simulink model "Traffic_Light_cs"  (R2019b)
settings: Solver=ode5  StartTime=0.0  StopTime=200  FixedStep=1/1000  RelTol=1e-3
PreLoadFcn:
  | mbxruntime.callbacks.PreLoadFcn(bdroot);
PostLoadFcn:
  | mbxruntime.callbacks.PostLoadFcn(bdroot);
InitFcn:
  | mbxruntime.callbacks.InitFcn(bdroot);
StartFcn:
  | mbxruntime.callbacks.StartFcn(bdroot);
StopFcn:
  | mbxruntime.callbacks.StopFcn(bdroot);
model workspace (MAT data in the model file):
  mbox_table : object (value not decoded)
  model_closed = 0
  sim_status = 0
values from neighbouring files (symbols this model uses):
  load_x1 = [-876.8956 -876.745665143 -876.595730285 -876.445795428 -876.29586057 -876.145925713 -875.995990855 -875.846055998 -875.69612114 -875.546186283 -875.396251425 -875.246316568 ... (5741 elements, 5741x1)]    [Data_ckx.mat]    (also in Load.mat)
  load_y1 = [537.3585 537.354079761 537.349659522 537.345239282 537.340819043 537.336398804 537.331978565 537.327558325 537.323138086 537.318717847 537.314297608 537.309877368 ... (5741 elements, 5741x1)]    [Data_ckx.mat]    (also in Load.mat)
  load_z1 = [0 0 0 0 0 0 0 0 0 0 0 0 ... (5741 elements, 5741x1)]    [Data_ckx.mat]    (also in Load.mat)
  q_pass = [0 0 0 37.0489514481 49.8894252687 51.0913174965 61.791576133 65.4762304223 75.669686677 80.4628164105 88.6197377629 94.2384891559 ... (437675 elements, 87535x5)]    [Data_ckx.mat]
  q_stop = [0 0 0 15.0544571491 15.7911831418 16.0935138936 18.6666396431 19.4721381181 21.7098800606 22.5642135149 25.0883481215 26.1253405703 ... (437675 elements, 87535x5)]    [Data_ckx.mat]
  s = roadinf.s    [Constraint_T_V.m]    (also in Light_Distinguish_old.m = 75:-0.7:75-84*0.7)
undefined symbols (not defined in the file or in its folder): InitImageOutputDir, mbxruntime, sigbuilder_block, tabledata
libraries: simulink x10, PreScanSimulinkLibrary x8, simulink_extras x4, autolibshared x1, fuzblock x1
(part 2 of 5)

== system Traffic_Light_cs/Synchronizer ==
  Bus Selector1 : BusSelector  OutputSignals=FederateStopped
  Stop Simulation : Stop
  sfun_Synchronizer : S-Function  FunctionName=sfun_Synchronizer  Parameters=SampleTime  SFunctionDeploymentMode=off  EnableBusSupport=off  mask(Legacy Function){SFunctionSpec=void prescan_synchronizer_outputFcn(void ** work1, PRESCAN_SYNCHRONIZEDATA y1[1]), SampleTime=TimeStep, ShowSpec=on}
      mask prompts: SampleTime "Sample time (-1 for inherited):"; ShowSpec "Display function specification"
      mask help:
      | This block allows you to call the legacy functions specified by the following Legacy Code Tool definition:
      | def.SFunctionName = 'sfun_Synchronizer';
      | def.OutputFcnSpec = 'void prescan_synchronizer_outputFcn(void ** work1, PRESCAN_SYNCHRONIZEDATA y1[1])';
      | def.StartFcnSpec = 'void prescan_synchronizer_startFcn(void ** work1)';
      | def.TerminateFcnSpec = 'void prescan_synchronizer_terminateFcn(void ** work1)';
      | def.HeaderFiles = {'prescan_synchronizer_data.h'};
      | def.HostLibFiles = {'sensorinterfaced.lib'};
      | def.IncPaths = {'src', 'C:\prescandev\vislibrary\vis\..\pimp\include\sensors\InterfaceRTW'};
      | def.SrcPaths = {'src'};
      | def.LibPaths = {'C:\\prescandev\\vislibrary_build\lib'};
      | def.SampleTime = 'parameterized';
      | def.Options.language = 'C';
      mask Help: <p>This block was generated automatically by the Legacy Code Tool. For detailed help on this tool, call<a href="matlab:legacy_code('help')"> legacy_code('help')</a>.</p>
      mask Callback ShowSpec:
      | if strcmp(get_param(gcbh, 'ShowSpec'), 'on')
      |   set_param(gcbh, 'MaskDisplay', sprintf('fprintf(''%s'');', get_param(gcbh, 'SFunctionSpec')));
      | else
      |   set_param(gcbh, 'MaskDisplay', sprintf('fprintf(''%s'');', get_param(gcbh, 'FunctionName')));
      | end
      mask Display: fprintf('void prescan_synchronizer_outputFcn(void ** work1, PRESCAN_SYNCHRONIZEDATA y1[1])');
  wires:
  Bus Selector1/1 -> Stop Simulation/1  "<FederateStopped>"
  sfun_Synchronizer/1 -> Bus Selector1/1

== system Traffic_Light_cs/VISUCasingLights_ID_1 ==
  VISUCasingLights_ID_1 : Inport  Tag=inport/VisuCasingLights  SampleTime=1/1000  BusOutputAsStruct=on
  Actuator : Subsystem  mask(PreScan Sink Block: VisuTrafficLight){UniqueID=35, ColorsObjectQuery=, Colors=[]}
      mask prompts: UniqueID "Parent Unique Identifier"; ColorsObjectQuery "Query for Color Object"; Colors "Matrix of colors"
      mask help:
      | The VisuTrafficLight block provides a way to animate traffic lights: switch on and off individual lights.
      |
      | For more information, please click Help.
      mask Help: eval('openHelp(731)')
      mask Display: image(imread('TrafficLightCasing.png'))
  wires:
  VISUCasingLights_ID_1/1 -> Actuator/1(VISUCasingLights_ID_1)

== system Traffic_Light_cs/VISUCasingLights_ID_2 ==
  VISUCasingLights_ID_2 : Inport  Tag=inport/VisuCasingLights  SampleTime=1/1000  BusOutputAsStruct=on
  Actuator : Subsystem  mask(PreScan Sink Block: VisuTrafficLight){UniqueID=525, ColorsObjectQuery=, Colors=[]}
      mask prompts: UniqueID "Parent Unique Identifier"; ColorsObjectQuery "Query for Color Object"; Colors "Matrix of colors"
      mask help:
      | The VisuTrafficLight block provides a way to animate traffic lights: switch on and off individual lights.
      |
      | For more information, please click Help.
      mask Help: eval('openHelp(731)')
      mask Display: image(imread('TrafficLightCasing.png'))
  wires:
  VISUCasingLights_ID_2/1 -> Actuator/1(VISUCasingLights_ID_2)

== system Traffic_Light_cs/VISUCasingLights_ID_3 ==
  VISUCasingLights_ID_3 : Inport  Tag=inport/VisuCasingLights  SampleTime=1/1000  BusOutputAsStruct=on
  Actuator : Subsystem  mask(PreScan Sink Block: VisuTrafficLight){UniqueID=526, ColorsObjectQuery=, Colors=[]}
      mask prompts: UniqueID "Parent Unique Identifier"; ColorsObjectQuery "Query for Color Object"; Colors "Matrix of colors"
      mask help:
      | The VisuTrafficLight block provides a way to animate traffic lights: switch on and off individual lights.
      |
      | For more information, please click Help.
      mask Help: eval('openHelp(731)')
      mask Display: image(imread('TrafficLightCasing.png'))
  wires:
  VISUCasingLights_ID_3/1 -> Actuator/1(VISUCasingLights_ID_3)

== system Traffic_Light_cs/CAR_Ahead/CameraSensor_2_CM_Demux ==
  In1 : Inport
  Selector : Selector  NumberOfDimensions=2  InputPortWidth=3  IndexOptions=Index vector (dialog),Index vector (dialog)  Indices=-1,1:hres  OutputSizes=1,1
  Selector1 : Selector  NumberOfDimensions=2  InputPortWidth=3  IndexOptions=Index vector (dialog),Index vector (dialog)  Indices=-1,hres+1:hres*2  OutputSizes=1,1
  Selector2 : Selector  NumberOfDimensions=2  InputPortWidth=3  IndexOptions=Index vector (dialog),Index vector (dialog)  Indices=-1,hres*2+1:hres*3  OutputSizes=1,1
  R : Outport
  G : Outport  Port=2
  B : Outport  Port=3
  wires:
  In1/1 -> Selector1/1, Selector/1, Selector2/1
  Selector/1 -> R/1
  Selector1/1 -> G/1
  Selector2/1 -> B/1

== system Traffic_Light_cs/CAR_Ahead/Decision ==
  Dis_Car2Light_Ahead : Inport
  CameraSensor_Ahead : Inport  Port=2
  Traffic_State : Inport  Port=3
  Traffic_Time : Inport  Port=4
  TrafficLight_ID_Ahead : Inport  Port=5
  PhaseTime : Inport  Tag=inport/SelfPort  Port=6  SampleTime=1/20  BusOutputAsStruct=on
  V_now : Inport  Port=7
  traffic_state : Inport  Port=8
  Bus Selector : BusSelector  OutputSignals=ID1,ID2,ID3
  Chart : Stateflow chart  TreatAsAtomicUnit=on
  Function-Call Subsystem : Subsystem  TreatAsAtomicUnit=on
  Multiport Switch : MultiPortSwitch  DiagnosticForDefault=None
  Light_State_Ahead : Outport  VectorParamsAs1DForOutWhenUnconnected=off
  TrafficLight_PhaseTime : Outport  Port=2  VectorParamsAs1DForOutWhenUnconnected=off
  wires:
  V_now/1 -> Function-Call Subsystem/5(V_now)
  Traffic_Time/1 -> Function-Call Subsystem/4(Traffic_Time)
  TrafficLight_ID_Ahead/1 -> Function-Call Subsystem/7(TrafficLight_ID_Ahead), Multiport Switch/1
  Chart/1(Decision_Call()) -> Function-Call Subsystem/Trigger
  Bus Selector/1 -> Multiport Switch/2  "<ID1>"
  Traffic_State/1 -> Function-Call Subsystem/3(Traffic_State)
  Bus Selector/2 -> Multiport Switch/3  "<ID2>"
  Function-Call Subsystem/1(Light_State_Ahead) -> Light_State_Ahead/1
  Bus Selector/3 -> Multiport Switch/4  "<ID3>"
  CameraSensor_Ahead/1 -> Function-Call Subsystem/2("CameraSensor ")
  Dis_Car2Light_Ahead/1 -> Chart/1(Dis_Car2Light_0919_100), Function-Call Subsystem/1(Dis)
  Multiport Switch/1 -> TrafficLight_PhaseTime/1
  PhaseTime/1 -> Bus Selector/1
  traffic_state/1 -> Function-Call Subsystem/6(traffic_state)

== system Traffic_Light_cs/CAR_Ahead/SELF_Demux ==
  SELF : Inport  OutDataTypeStr=Bus: PRESCAN_SELFSENSORDATA
  Bus Selector : BusSelector  OutputSignals=PositionX,PositionY,PositionZ,OrientationRoll,OrientationPitch,OrientationYaw,Velocity,Yaw_rate,Lat,Long,Alt
  Demux2 : Demux  Outputs=3
  Gain : Gain  Gain=180/pi
  Gain1 : Gain  Gain=180/pi
  Vector Concatenate1 : Concatenate  NumInputs=3
  compas converter : Subsystem
  x [m] : Outport
  y [m] : Outport  Port=2
  z [m] : Outport  Port=3
  rotx [deg] : Outport  Port=4
  roty [deg] : Outport  Port=5
  rotz [deg] : Outport  Port=6
  GPS lat [deg] : Outport  Port=7
  GPS long [deg] : Outport  Port=8
  GPS alt [m] : Outport  Port=9
  velocity [m/s] : Outport  Port=10
  heading [deg] : Outport  Port=11
  yaw rate [deg/s] : Outport  Port=12
  wires:
  Bus Selector/11 -> GPS alt [m]/1  "<Alt>"
  Bus Selector/10 -> GPS long [deg]/1  "<Long>"
  Bus Selector/9 -> GPS lat [deg]/1  "<Lat>"
  Bus Selector/8 -> Gain1/1  "<Yaw_rate>"
  Bus Selector/7 -> velocity [m/s]/1  "<Velocity>"
  Bus Selector/6 -> compas converter/1(rotz [rad]), Vector Concatenate1/3  "<OrientationYaw>"
  Bus Selector/5 -> Vector Concatenate1/2  "<OrientationPitch>"
  Bus Selector/4 -> Vector Concatenate1/1  "<OrientationRoll>"
  Vector Concatenate1/1 -> Gain/1
  Bus Selector/3 -> z [m]/1  "<PositionZ>"
  Bus Selector/2 -> y [m]/1  "<PositionY>"
  Bus Selector/1 -> x [m]/1  "<PositionX>"
  SELF/1 -> Bus Selector/1
  Gain/1 -> Demux2/1
  Demux2/1 -> rotx [deg]/1
  Demux2/2 -> roty [deg]/1
  Demux2/3 -> rotz [deg]/1
  compas converter/1(heading [deg]) -> heading [deg]/1
  Gain1/1 -> yaw rate [deg/s]/1

== system Traffic_Light_cs/CAR_Ahead/STATE_CAR_Ahead ==
  State : Inport  SampleTime=TimeStep
  Bus Creator : BusCreator  Inputs=15  OutDataTypeStr=Bus: PRESCAN_STATEACTUATORDATA  NonVirtualBus=on
  Demux : Demux  Outputs=15
  iniBODYAngles wrtVEH [rad] : Constant  Value=[Roll0 Pitch0 0]  SampleTime=TimeStep
  iniVEHAngles wrtGLOB [rad] : Constant  Value=[0 0 Yaw0]  SampleTime=TimeStep
  iniVEHposition wrtGLOB [m] : Constant  Value=[x0 y0 z0]  SampleTime=TimeStep
  state2FullState : PreScanSimulinkLibrary/state2FullState  SystemSampleTime=-1  Latency=0  AutoFrameSizeCalculation=off
  StateBus : Outport  OutDataTypeStr=Bus: PRESCAN_STATEACTUATORDATA
  wires:
  Bus Creator/1 -> StateBus/1
  State/1 -> state2FullState/1
  state2FullState/1 -> Demux/1
  iniVEHposition wrtGLOB [m]/1 -> state2FullState/2
  iniBODYAngles wrtVEH [rad]/1 -> state2FullState/3
  iniVEHAngles wrtGLOB [rad]/1 -> state2FullState/4
  Demux/1 -> Bus Creator/1  "PositionX"
  Demux/2 -> Bus Creator/2  "PositionY"
  Demux/3 -> Bus Creator/3  "PositionZ"
  Demux/4 -> Bus Creator/4  "VelocityX"
  Demux/5 -> Bus Creator/5  "VelocityY"
  Demux/6 -> Bus Creator/6  "VelocityZ"
  Demux/7 -> Bus Creator/7  "AccelerationX"
  Demux/8 -> Bus Creator/8  "AccelerationY"
  Demux/9 -> Bus Creator/9  "AccelerationZ"
  Demux/10 -> Bus Creator/10  "OrientationRoll"
  Demux/11 -> Bus Creator/11  "OrientationPitch"
  Demux/12 -> Bus Creator/12  "OrientationYaw"
  Demux/13 -> Bus Creator/13  "AngularVelocityRoll"
  Demux/14 -> Bus Creator/14  "AngularVelocityPitch"
  Demux/15 -> Bus Creator/15  "AngularVelocityYaw"

== system Traffic_Light_cs/CAR_Ahead/Subsystem ==
  x [m] : Inport
  y [m] : Inport  Port=2
  Bus Creator : BusCreator  Inputs=6
  Bus Creator1 : BusCreator  Inputs=4
  Delay : Delay
  Delay1 : Delay
  MATLAB Function : MATLAB Function  TreatAsAtomicUnit=on
  Signal Builder : Subsystem  Tag=STV Subsys  LoadFcn=sigbuilder_block('load');  StartFcn=sigbuilder_block('start');  StopFcn=sigbuilder_block('stop');  ClipboardFcn=sigbuilder_block('clipboard');  mask(Sigbuilder block){tuvar=[0:10]}
      mask help: Simulink:masks:SigbuilderBlock_MD
      mask init:
      | if ~strcmp(get_param(bdroot(gcbh),'SimulationStatus'),'stopped') tuvar = sigbuilder_block('maskInit'); end
      settings: CopyFcn=sigbuilder_block('copy');  DeleteFcn=sigbuilder_block('delete');  ModelCloseFcn=sigbuilder_block('modelClose');  PreSaveFcn=sigbuilder_block('preSave');  PauseFcn=sigbuilder_block('pause');  ContinueFcn=sigbuilder_block('continue');  NameChangeFcn=sigbuilder_block('namechange');  OpenFcn=sigbuilder_block('open',[6 6 1188 604.5 ]);  CloseFcn=sigbuilder_block('close');
      mask Display: plot(0, 0, 100, 100,[2, 2, 32, 32, 2], [68, 8, 8, 68, 68],[32, 2], [38, 38], [32, 19, 2],[53, 60, 44], [32, 17, 17, 2],[16, 16, 31, 31]);txt = getActiveGroup(gcbh);text(2, 100, txt,'verticalAlignment', 'top');
  Distance2Light : Outport  VectorParamsAs1DForOutWhenUnconnected=off
  TrafficLight_ID : Outport  Port=2  VectorParamsAs1DForOutWhenUnconnected=off
  wires:
  MATLAB Function/2(Dis_Car2Light) -> Distance2Light/1  "Dis_Car2Light"
  Bus Creator1/1 -> MATLAB Function/1(Car_GPS)
  Delay/1 -> Bus Creator1/3
  Delay1/1 -> Bus Creator1/1
  MATLAB Function/1(TrafficLight_ID) -> TrafficLight_ID/1  "TrafficLight_ID"
  Bus Creator/1 -> MATLAB Function/2(TrafficLight_GPS)
  Signal Builder/6(ID==3,Y) -> Bus Creator/6
  Signal Builder/5(ID==3,X) -> Bus Creator/5
  Signal Builder/4(ID==2,Y) -> Bus Creator/4
  Signal Builder/3(ID==2,X) -> Bus Creator/3
  Signal Builder/2(ID==1,Y) -> Bus Creator/2
  Signal Builder/1(ID==1,X) -> Bus Creator/1
  y [m]/1 -> Bus Creator1/4, Delay/1
  x [m]/1 -> Bus Creator1/2, Delay1/1

== system Traffic_Light_cs/CAR_Ahead/Trajectories ==
  Traj2State1 : Subsystem  Tag=Traj2State  mask(PreScan Demux Block:){}
      settings: DeleteFcn=PreScanBlockDeleteFcn;
  TrajCoGOffset : Subsystem  Tag=TrajCoGOffset  mask(Trajectory CoG Offset block){CoGOffsetZ=0.55, InitRoll=0, InitPitch=0}
      mask prompts: CoGOffsetZ "Z-component of CoG Offset [m]:"; InitRoll "Initial Roll angle [deg]:"; InitPitch "Initial Pitch angle [deg]:"
      mask help: A trajectory follows the surface of the road. However the position of a actor is based on the actor's Center of Gravity, which is typically above the road. This block converts from the trajectory along the road surface to the trajectory of the actor's CoG by realigning the z-component of the CoG offset to be normal to the road.
      settings: DeleteFcn=PreScanBlockDeleteFcn;
  Trajectory_1 : Subsystem  Tag=Trajectory  mask(PreScan Source Block: Trajectory){FileName='Trajectory_1.mat', TimeStep=1/1000}
      mask prompts: TimeStep "Time Step [s]"
      mask help:
      | The Trajectory block contains the trajectories defined in the PreScan Experiment Editor. The output of the trajectory block is the (vehicle) State.
      |
      | For more information, please click Help.
      mask init:
      | EXPROOT=pwd;  % TODO better construction for locating base experiment
      | 
      | trajfilename = fullfile(EXPROOT,'Trajectories',FileName);
      | load(trajfilename);
      | trajectory=trajectory';
      | 
      | traj.time=trajectory(:,1);%[];
      | traj.signals.values=trajectory(:,2:19);
      | traj.dimensions=18;
      | traj.label='';
      | 
      | SampleTime=traj.time(2)-traj.time(1);
      settings: DeleteFcn=PreScanBlockDeleteFcn;
      mask Help: eval('openHelp(312)')
      mask Display: fprintf(FileName)
  Trajectory_1_Offset : Constant  Tag=TrajectoryOffset  Value="[0  0  0  0  0  0]"
  State : Outport  Tag=TrajOutport
  wires:
  Trajectory_1/1(trajectory) -> Traj2State1/1(Traj Org)
  Trajectory_1_Offset/1 -> Traj2State1/2(Offset)
  TrajCoGOffset/1(State Out) -> State/1
  Traj2State1/1(state) -> TrajCoGOffset/1(State In)

== system Traffic_Light_cs/CAR_Ahead/V2V_Output ==
  Traffic_State : Inport
  Dis_Car2Light_Ahead : Inport  Port=2
  Light_State_Ahead : Inport  Port=3
  TrafficLight_ID_Ahead : Inport  Port=4
  Traffic_Time : Inport  Port=5
  TrafficLight_PhaseTime : Inport  Port=6
  Bus Creator : BusCreator  Inputs=3
  Switch : Switch  Criteria=u2 > Threshold
  Switch1 : Switch  Criteria=u2 > Threshold  Threshold=500
  Traffic_Information : Outport  VectorParamsAs1DForOutWhenUnconnected=off
  "Traffic_Time " : Outport  Port=2  VectorParamsAs1DForOutWhenUnconnected=off
  wires:
  Light_State_Ahead/1 -> Switch1/3
  Bus Creator/1 -> Traffic_Information/1
  Traffic_State/1 -> Switch1/1
  TrafficLight_PhaseTime/1 -> Switch/3
  Switch1/1 -> Bus Creator/1  "LightState_Ahead"
  TrafficLight_ID_Ahead/1 -> Bus Creator/2  "ID_Ahead"
  Traffic_Time/1 -> Switch/1, Switch/2
  Dis_Car2Light_Ahead/1 -> Switch1/2
  Switch/1 -> Bus Creator/3, "Traffic_Time "/1  "TrafficTime_Ahead"

== system Traffic_Light_cs/CAR_Main/CameraSensor_1_CM_Demux ==
  In1 : Inport
  Selector : Selector  NumberOfDimensions=2  InputPortWidth=3  IndexOptions=Index vector (dialog),Index vector (dialog)  Indices=-1,1:hres  OutputSizes=1,1
  Selector1 : Selector  NumberOfDimensions=2  InputPortWidth=3  IndexOptions=Index vector (dialog),Index vector (dialog)  Indices=-1,hres+1:hres*2  OutputSizes=1,1
  Selector2 : Selector  NumberOfDimensions=2  InputPortWidth=3  IndexOptions=Index vector (dialog),Index vector (dialog)  Indices=-1,hres*2+1:hres*3  OutputSizes=1,1
  R : Outport
  G : Outport  Port=2
  B : Outport  Port=3
  wires:
  In1/1 -> Selector1/1, Selector/1, Selector2/1
  Selector/1 -> R/1
  Selector1/1 -> G/1
  Selector2/1 -> B/1

== system Traffic_Light_cs/CAR_Main/Decision ==
  Dis_Car2Light_Main : Inport
  CameraSensor_Main : Inport  Port=2
  Traffic_State : Inport  Port=3
  Traffic_Time : Inport  Port=4
  TrafficLight_ID_Main : Inport  Port=5
  PhaseTime : Inport  Tag=inport/SelfPort  Port=6  SampleTime=1/20  BusOutputAsStruct=on
  V_now : Inport  Port=7
  traffic_state : Inport  Port=8
  Bus Selector : BusSelector  OutputSignals=ID1,ID2,ID3
  Chart : Stateflow chart  TreatAsAtomicUnit=on
  Function-Call Subsystem : Subsystem  TreatAsAtomicUnit=on
  Multiport Switch : MultiPortSwitch  DiagnosticForDefault=None
  Switch : Switch  Criteria=u2 > Threshold  Threshold=-1
  Transfer Fcn : TransferFcn  Denominator=[4 1]
  Light_State_Main : Outport  VectorParamsAs1DForOutWhenUnconnected=off
  TrafficLight_PhaseTime : Outport  Port=2  VectorParamsAs1DForOutWhenUnconnected=off
  V_Target : Outport  Port=3  VectorParamsAs1DForOutWhenUnconnected=off
  wires:
  Transfer Fcn/1 -> Switch/3
  Function-Call Subsystem/2(V_Target) -> Switch/1, Transfer Fcn/1
  Switch/1 -> V_Target/1
  Function-Call Subsystem/3("Suggest ") -> Switch/2
  V_now/1 -> Function-Call Subsystem/5(V_now)
  Traffic_Time/1 -> Function-Call Subsystem/4(Traffic_Time)
  TrafficLight_ID_Main/1 -> Function-Call Subsystem/7(TrafficLight_ID_Main), Multiport Switch/1
  Chart/1(Decision_Call()) -> Function-Call Subsystem/Trigger
  Bus Selector/3 -> Multiport Switch/4  "<ID3>"
  Bus Selector/1 -> Multiport Switch/2  "<ID1>"
  Traffic_State/1 -> Function-Call Subsystem/3(Traffic_State)
  Bus Selector/2 -> Multiport Switch/3  "<ID2>"
  Function-Call Subsystem/1(Light_State_Main) -> Light_State_Main/1
  CameraSensor_Main/1 -> Function-Call Subsystem/2("CameraSensor ")
  Dis_Car2Light_Main/1 -> Chart/1(Dis_Car2Light_0919_100), Function-Call Subsystem/1(Dis)
  Multiport Switch/1 -> TrafficLight_PhaseTime/1
  PhaseTime/1 -> Bus Selector/1
  traffic_state/1 -> Function-Call Subsystem/6(traffic_state)

== system Traffic_Light_cs/CAR_Main/Driver Model ==
  VehSpdTarKph : Inport
  VehSpdActKph : Inport  Port=2
  Grade[deg] : Inport  Port=3
  Abs : Abs
  Compare To Constant : simulink/Logic and Bit Operations/Compare To Constant  relop=<=  const=2/3.6  OutDataTypeStr=boolean
  Compare To Zero : simulink/Logic and Bit Operations/Compare To Zero  relop===  OutDataTypeStr=boolean
  Compare To Zero2 : simulink/Logic and Bit Operations/Compare To Zero  relop=>=  OutDataTypeStr=boolean
  Constant : Constant  Value=20
  D : Constant  Value=3
  Gain3 : Gain  Gain=100
  Gain4 : Gain  Gain=100
  Logical Operator : Logic  AllPortsSameDT=off  OutDataTypeStr=boolean
  Longitudinal Driver : autolibshared/Longitudinal Driver  cntrlType=PI  shftType=None  velUnits=m/s  gearOut=off  Kp=5  Ki=3  Kff=.01  Kg=.01  VehVelVec=[0 100]  KffVec=[.1 .1]  KpVec=[10 10]  KiVec=[5 5]  KgVec=[0 0]  m=1500  Kpt=3000  tau=.1  L=2  aR=200  bR=2.5  cR=.5  g=9.81  vnom=60  Kaw=.1  tauerr=.03  tauPt=2  GearInit=0  tShift=.1  pdlVec=[0.1 0.4 0.5 0.9]  upShftTbl=[-1 12.9375 26.4375 39.9375 51.18749999999999 62.4375 72.84375 83.25;-1 16.3125 29.8125 43.3125 54.5624 65.8125 76.78125 87.75;-1 19.6875 33.1875 46.68749999999999 57.9375 69.1875 80.71875 92.25;-1 33 52.5 77.25 100.5 138.75 161.875 185]  dwnShftTbl=[1 9.5625 23.0625 36.5625 47.8125 59.0625 68.90625 78.75;1 12.9375 26.4375 39.9375 51.18749999999999 62.4375 72.84375 83.25;1 16.3125 29.8125 43.3125 54.562499 65.8125 76.78125 87.75;1 19.6875 33.1875 46.68749999999999 57.9375 69.1875 80.71875 92.25]  tClutch=.5  tRev=.5  tPark=120  aMode=1  UpGearVec="[0  1  2  3  4  5  6  7]"  DownGearVec="[1  2  3  4  5  6  7  8]"
      settings: SourceProductBaseCode=PW
  N : Constant  Value=2
  R : Constant
  Relational Operator : RelationalOperator  Operator=~=  OutDataTypeStr=boolean  RndMeth=Simplest
  Subtract : Sum  Inputs=+-
  Switch1 : Switch  Criteria=u2 > Threshold
  Switch2 : Switch  Criteria=u2 > Threshold
  Switch3 : Switch  Criteria=u2 ~= 0
  Terminator : Terminator
  AccPedlRat% : Outport  VectorParamsAs1DForOutWhenUnconnected=off
  BrkPedlRat% : Outport  Port=2  VectorParamsAs1DForOutWhenUnconnected=off
  ShiftLvr : Outport  Port=3  VectorParamsAs1DForOutWhenUnconnected=off
  wires:
  Longitudinal Driver/1 -> Terminator/1
  Abs/1 -> Compare To Constant/1
  Subtract/1 -> Abs/1
  Constant/1 -> Switch3/3
  Gain4/1 -> Switch3/1  "BrkPedl"
  Relational Operator/1 -> Switch3/2
  R/1 -> Switch2/3
  Compare To Zero2/1 -> Switch2/2
  D/1 -> Switch2/1
  Compare To Constant/1 -> Logical Operator/2
  Compare To Zero/1 -> Logical Operator/1
  Logical Operator/1 -> Switch1/2
  Switch3/1 -> BrkPedlRat%/1  "BrkPedl"
  Longitudinal Driver/2 -> Gain3/1
  Longitudinal Driver/3 -> Gain4/1
  VehSpdTarKph/1 -> Compare To Zero/1, Compare To Zero2/1, Subtract/1, Longitudinal Driver/1
  Grade[deg]/1 -> Longitudinal Driver/3
  VehSpdActKph/1 -> Subtract/2, Longitudinal Driver/2
  Switch2/1 -> Switch1/3
  Switch1/1 -> ShiftLvr/1, Relational Operator/2
  N/1 -> Relational Operator/1, Switch1/1
  Gain3/1 -> AccPedlRat%/1  "AccPedl"

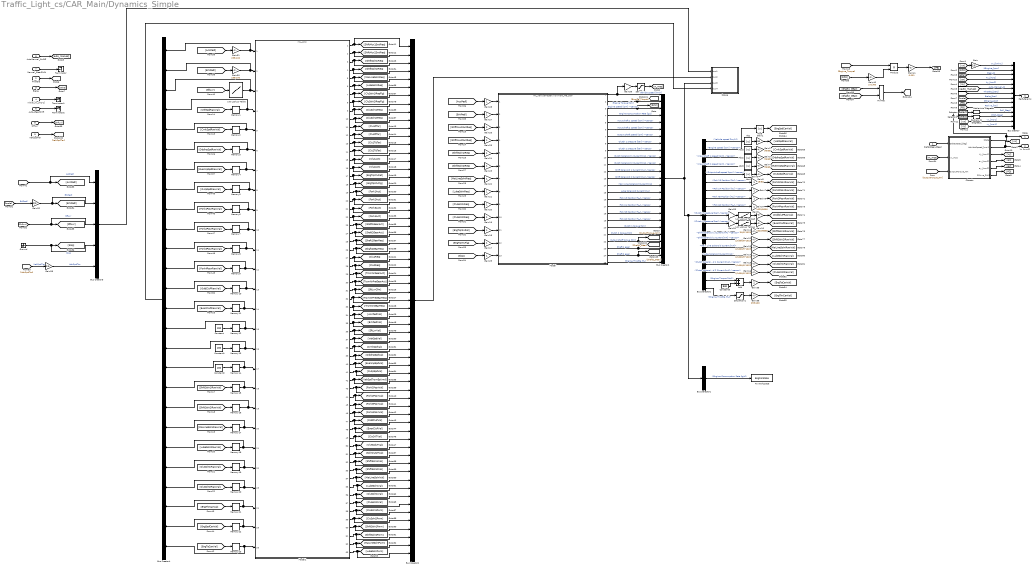
== system Traffic_Light_cs/CAR_Main/Dynamics_Simple ==
  DeltaSteer_[deg] : Inport
  Throttle : Inport  Port=2
  Brake : Inport  Port=3
  Initial_Vx_[ms-1] : Inport  Port=4
  AutoManual_OnOff : Inport  Port=5
  Auto_GearShift : Inport  Port=6
  Manual_GearShift : Inport  Port=7
  "ShfLvr " : Inport  Port=8
  "VehSpdTar " : Inport  Port=9
  1-D Lookup Table : Lookup_n-D  NumberOfTableDimensions=1  BreakpointsForDimension1=[0 1 2 3]  Table=[8 7 6 5]  TableDataTypeStr=uint8  InterpMethod=Flat  ExtrapMethod=Clip  DiagnosticForOutOfRangeInput=Warning  InternalRulePriority=Speed  OutDataTypeStr=uint8  RndMeth=Simplest  InputSameDT=on
  1-D Lookup Table1 : Lookup_n-D  NumberOfTableDimensions=1  BreakpointsForDimension1=[310,2500,20000]  Table=[0,500,4500]  TableDataTypeStr=Inherit: Inherit from 'Table data'  ExtrapMethod=Clip  UseLastTableValue=on  InternalRulePriority=Speed  OutDataTypeStr=Inherit: Inherit from 'Table data'  RndMeth=Simplest  InputSameDT=on
  1-D Lookup Table3 : Lookup_n-D  NumberOfTableDimensions=1  BreakpointsForDimension1=[310,2500,20000]  Table=[0,500,4500]  TableDataTypeStr=Inherit: Inherit from 'Table data'  ExtrapMethod=Clip  UseLastTableValue=on  InternalRulePriority=Speed  OutDataTypeStr=Inherit: Inherit from 'Table data'  RndMeth=Simplest  InputSameDT=on
  Abs{,1..4} (5 alike) : Abs
  Abs5 : Abs  OutDataTypeStr=uint16
  Add : Sum
  Bus Creator : BusCreator  Inputs=14
  Bus Creator1 : BusCreator  Inputs=25
  Bus Creator2 : BusCreator  Inputs=63
  Bus Creator3 : BusCreator  Inputs=5
  Bus Creator4 : BusCreator  Inputs=26
  Bus Selector1 : BusSelector  OutputSignals=Engine Consumption Rate [g/s]
  Bus Selector2 : BusSelector  OutputSignals=Vehicle speed [km/h],Engine speed [rpm] ->sensor,Input shaft 1 speed [rpm] ->sensor,Input shaft 2 speed [rpm] ->sensor,Output shaft speed [rpm] ->sensor,Fork 13 Position [‰] ->sensor,Fork 24 Position [‰] ->sensor,Fork N5 Position [‰] ->sensor,Fork 6R Position [‰] ->sensor,Clutch 1 pressure [bar] ->sensor,Clutch 2 pressure [bar] ->sensor,Shift Solenoid 1 Current [mA] ->sensor,Shift Solenoid 2 Current [mA] ->sensor,Main Line Solenoid Current [mA],Lube Solenoid Current [mA],Clutch Solenoid 1 Current [mA] ->sensor,Clutch Solenoid 2 Current [mA] ->sensor,Engine Torque [Nm],Engine Throttle [%]
  Chassis : Subsystem
      mask Display: image(imread('Chassis.png'));
  Constant : Constant  Value=200  OutDataTypeStr=uint16
  Constant1 : Constant  Value=200  OutDataTypeStr=uint16
  Constant2 : Constant  Value=200  OutDataTypeStr=uint16
  Constant3 : Constant  Value=848
  Gain : Gain  Gain=3.6
  Gain1 : Gain  Gain=64  OutDataTypeStr=uint16
  Gain10 : Gain  Gain=1023/5000  OutDataTypeStr=uint16
  Gain{11..16} (6 alike) : Gain  Gain=2/1000/5*1023  OutDataTypeStr=uint16
  Gain{17..29} (13 alike) : Gain  OutDataTypeStr=double
  Gain2 : Gain  Gain=36/60  OutDataTypeStr=uint16
  Gain3 : Gain  Gain=36/60  OutDataTypeStr=uint16
  Gain30 : Gain  Gain=255/100  OutDataTypeStr=uint8
  Gain31 : Gain  Gain=255/100  OutDataTypeStr=uint8
  Gain32 : Gain  Gain=2/3
  Gain33 : Gain  Gain=1000  OutDataTypeStr=uint16
  Gain34 : Gain  Gain=1000  OutDataTypeStr=uint16
  Gain35 : Gain  Gain=2  OutDataTypeStr=uint16
  Gain36 : Gain  Gain=255/100  OutDataTypeStr=uint8
  Gain37 : Gain  Gain=1023/5000  OutDataTypeStr=uint16
  Gain38 : Gain  Gain=3.6
  Gain39 : Gain  Gain=1/3.6
  Gain4 : Gain  Gain=36/60  OutDataTypeStr=uint16
  Gain40 : Gain  Gain=2*pi/60
  Gain41 : Gain  Gain=0.001
  Gain5 : Gain  Gain=18/60  OutDataTypeStr=uint16
  Gain{6..9} (4 alike) : Gain  OutDataTypeStr=uint16
  Ground : Ground
  Memory{1..23} (23 alike) : Memory  InheritSampleTime=on
  MinMax : MinMax  Function=max  Inputs=2
  Model : ModelReference  ModelNameDialog=MIL_VehicleTestEnvironment_MG_DCT.mdl  SimulationMode=Normal  ModelReferenceVersion=1.244
  Model1 : ModelReference  ModelNameDialog=MIL_ASW.slx  SimulationMode=Normal  ModelReferenceVersion=1.234
  Product : Product
  Radians to Degrees : simulink_extras/Transformations/Radians to Degrees
  Radians to Degrees1 : simulink_extras/Transformations/Radians to Degrees
  Saturation : Saturate  UpperLimit=20  LowerLimit=0
  Saturation1 : Saturate  UpperLimit=100  LowerLimit=0  OutDataTypeStr=double
  Scope : Subsystem
  Selector : Selector  InputPortWidth=9  IndexOptions=Index vector (dialog)  Indices=7  OutputSizes=1
  Selector1 : Selector  InputPortWidth=9  IndexOptions=Index vector (dialog)  Indices=8  OutputSizes=1
  Terminator : Terminator
  Terminator1 : Terminator
  Terminator2 : Terminator
  To Workspace : ToWorkspace  VariableName=EngConRate  SaveFormat=Timeseries  SampleTime=-1
  State : Outport  VectorParamsAs1DForOutWhenUnconnected=off
  Vx [m s-1] : Outport  Port=2  VectorParamsAs1DForOutWhenUnconnected=off
  Perf_Params : Outport  Port=3  VectorParamsAs1DForOutWhenUnconnected=off
  wires:
  Saturation/1 -> [vx_mps]
  Auto_GearShift/1 -> Terminator2/1
  Initial_Vx_[ms-1]/1 -> Terminator1/1
  Manual_GearShift/1 -> Terminator/1
  MinMax/1 -> [gear]
  [Shaft2_Gear] -> MinMax/2
  [Shaft1_Gear] -> MinMax/1
  Gain40/1 -> Product/2
  Gain41/1 -> [PE]
  [Engine_Torque] -> Product/1
  Product/1 -> Gain41/1
  [RPM] -> Gain40/1
  [OutputTorque_Nm] -> Chassis/3(OutputTorque_Nm)
  [vx_mps] -> Chassis/2(vx_mps)
  DeltaSteer_[deg]/1 -> Chassis/1(DeltaSteer_[deg])
  Brake/1 -> [brake]
  Throttle/1 -> [throttle]
  AutoManual_OnOff/1 -> [auto_manual]
  "ShfLvr "/1 -> [ShfLvr]
  "VehSpdTar "/1 -> [VehSpdTar]
  Gain39/1 -> Saturation/1
  Gain38/1 -> Bus Creator3/5  "VehSpdTar"
  Gain32/1 -> Bus Creator3/2, [BrkPedl]  "BrkPedl"
  Model/24 -> Bus Creator1/24, [Shaft2_Gear]  "Shaft 2 gear"
  Model/1 -> Gain39/1, Bus Creator1/1  "Vehicle speed [km/h]"
  Model/2 -> Bus Creator1/2, [Engine_Torque]  "Engine Torque [Nm]"
  Model/15 -> Bus Creator1/15  "Lube Solenoid Current [mA]"
  Model/23 -> Bus Creator1/23, [Shaft1_Gear]  "Shaft 1 gear"
  Model/19 -> Bus Creator1/19  "Fork 6R Position [‰] ->sensor"
  Model/5 -> Bus Creator1/5  "Input shaft 1 speed [rpm] ->sensor"
  Model/10 -> Bus Creator1/10  "Clutch Solenoid 1 Current [mA] ->sensor"
  Model/20 -> Bus Creator1/20  "Clutch 1 torque [Nm]"
  Model/9 -> Bus Creator1/9  "Clutch 2 pressure [bar] ->sensor"
  Model/3 -> Bus Creator1/3, [RPM]  "Engine speed [rpm] ->sensor"
  Model/14 -> Bus Creator1/14  "Main Line Solenoid Current [mA]"
  Model/12 -> Bus Creator1/12  "Shift Solenoid 1 Current [mA] ->sensor"
  Model/22 -> Bus Creator1/22, [OutputTorque_Nm]  "Output shaft torque [Nm]"
  Model/16 -> Bus Creator1/16  "Fork 13 Position [‰] ->sensor"
  Model/8 -> Bus Creator1/8  "Clutch 1 pressure [bar] ->sensor"
  Model/17 -> Bus Creator1/17  "Fork 24 Position [‰] ->sensor"
  Model/6 -> Bus Creator1/6  "Input shaft 2 speed [rpm] ->sensor"
  Model/11 -> Bus Creator1/11  "Clutch Solenoid 2 Current [mA] ->sensor"
  Model/13 -> Bus Creator1/13  "Shift Solenoid 2 Current [mA] ->sensor"
  Model/18 -> Bus Creator1/18  "Fork N5 Position [‰] ->sensor"
  Model/21 -> Bus Creator1/21  "Clutch 2 torque [Nm]"
  Model/7 -> Bus Creator1/7  "Output shaft speed [rpm] ->sensor"
  Model1/1 -> Bus Creator2/1, [ShiftMux1SwtReq]
  Model1/2 -> Bus Creator2/2, [ShiftMux2SwtReq]
  Model1/20 -> Bus Creator2/20, [Fork2Act]
  Model1/13 -> Bus Creator2/13, [Clu1TqTar]
  Model1/21 -> Bus Creator2/21, [Fork3Act]
  Model1/22 -> Bus Creator2/22, [Fork4Act]
  Model1/23 -> Bus Creator2/23, [Shaft1GearAct]
  Model1/4 -> Bus Creator2/4, [ShiftSoln2IReq]
  Model1/3 -> Bus Creator2/3, [ShiftSoln1IReq]
  Model1/7 -> Bus Creator2/7, [CluSoln1IReqFlg]
  Model1/9 -> Bus Creator2/9, [CluSoln1IReq]
  Model1/15 -> Bus Creator2/15, [Clu1Act]
  Model1/16 -> Bus Creator2/16, [Clu2Act]
  Model1/8 -> Bus Creator2/8, [CluSoln2IReqFlg]
  Model1/14 -> Bus Creator2/14, [Clu2TqTar]
  Model1/17 -> Bus Creator2/17, [EngTqIntvRat]
  Model1/6 -> Bus Creator2/6, [LubeSolnIReq]
  Model1/11 -> Bus Creator2/11, [Clu1PTar]
  Model1/5 -> Bus Creator2/5, [MaiLineSolnIReq]
  Model1/10 -> Bus Creator2/10, [CluSoln2IReq]
  Model1/12 -> Bus Creator2/12, [Clu2PTar]
  Model1/18 -> Bus Creator2/18, [EngTqIntvFlg]
  Model1/19 -> Bus Creator2/19, [Fork1Act]
  Model1/27 -> Bus Creator2/27, [Clu1Req]
  Model1/25 -> Bus Creator2/25, [Shaft1GearReq]
  Model1/28 -> Bus Creator2/28, [Clu2Req]
  Model1/24 -> Bus Creator2/24, [Shaft2GearAct]
  Model1/26 -> Bus Creator2/26, [Shaft2GearReq]
  Model1/29 -> Bus Creator2/29, [TrsmNrGearAct]
  Model1/30 -> Bus Creator2/30, [TrsmNrPreGearAct]
  Model1/32 -> Bus Creator2/32, [TrsmNrPreGearReq]
  Model1/33 -> Bus Creator2/33, [TrsmNrGearReq]
  Model1/35 -> Bus Creator2/35, [BrkPedlVal]
  Model1/31 -> Bus Creator2/31, [SftLvrCfm]
  Model1/34 -> Bus Creator2/34, [AccPedlVal]
  Model1/36 -> Bus Creator2/36, [SftLvrVal]
  Model1/37 -> Bus Creator2/37, [VehSpdVal]
  Model1/38 -> Bus Creator2/38, [CrnkSpdVal]
  Model1/39 -> Bus Creator2/39, [OddInpSpdVal]
  Model1/40 -> Bus Creator2/40, [EvenInpSpdVal]
  Model1/41 -> Bus Creator2/41, [OutpSpdVal]
  Model1/52 -> Bus Creator2/52, [ShiftSoln1IVal]
  Model1/55 -> Bus Creator2/55, [LubeSolnIVal]
  Model1/45 -> Bus Creator2/45, [Fork3PosnVal]
  Model1/49 -> Bus Creator2/49, [CluOilTVal]
  Model1/48 -> Bus Creator2/48, [EvenCluPVal]
  Model1/53 -> Bus Creator2/53, [ShiftSoln2IVal]
  Model1/54 -> Bus Creator2/54, [MaiLineSolnIVal]
  Model1/56 -> Bus Creator2/56, [CluSoln1IVal]
  Model1/47 -> Bus Creator2/47, [OddCluPVal]
  Model1/57 -> Bus Creator2/57, [CluSoln2IVal]
  Model1/42 -> Bus Creator2/42, [VehSpdTrsmEstimd]
  Model1/43 -> Bus Creator2/43, [Fork1PosnVal]
  Model1/44 -> Bus Creator2/44, [Fork2PosnVal]
  Model1/46 -> Bus Creator2/46, [Fork4PosnVal]
  Model1/50 -> Bus Creator2/50, [VlvBodyTVal]
  Model1/51 -> Bus Creator2/51, [SolnOutpTVal]
  Bus Selector2/1 -> Abs/1  "<Vehicle speed [km/h]>"
  Bus Selector2/2 -> Abs5/1, Abs1/1  "<Engine speed [rpm] ->sensor>"
  Gain1/1 -> [VehSpdRawVal]
  Gain2/1 -> [CrnkSpdRawVal]
  Bus Selector2/3 -> Abs2/1  "<Input shaft 1 speed [rpm] ->sensor>"
  Bus Selector2/4 -> Abs3/1  "<Input shaft 2 speed [rpm] ->sensor>"
  Bus Selector2/5 -> Abs4/1  "<Output shaft speed [rpm] ->sensor>"
  Gain3/1 -> [OddInpSpdRawVal]
  Gain4/1 -> [EvenInpSpdRawVal]
  Gain5/1 -> [OutpSpdRawVal]
  Bus Selector2/6 -> Gain6/1  "<Fork 13 Position [‰] ->sensor>"
  Bus Selector2/8 -> Gain8/1  "<Fork N5 Position [‰] ->sensor>"
  Bus Selector2/9 -> Gain9/1  "<Fork 6R Position [‰] ->sensor>"
  Bus Selector2/7 -> Gain7/1  "<Fork 24 Position [‰] ->sensor>"
  Bus Selector2/10 -> Gain33/1  "<Clutch 1 pressure [bar] ->sensor>"
  Bus Selector2/11 -> Gain34/1  "<Clutch 2 pressure [bar] ->sensor>"
  Bus Selector2/16 -> Gain15/1  "<Clutch Solenoid 1 Current [mA] ->sensor>"
  Bus Selector2/13 -> Gain12/1  "<Shift Solenoid 2 Current [mA] ->sensor>"
  Bus Selector2/15 -> Gain14/1  "<Lube Solenoid Current [mA]>"
  Bus Selector2/14 -> Gain13/1  "<Main Line Solenoid Current [mA]>"
  Bus Selector2/17 -> Gain16/1  "<Clutch Solenoid 2 Current [mA] ->sensor>"
  Bus Selector2/12 -> Gain11/1  "<Shift Solenoid 1 Current [mA] ->sensor>"
  Gain7/1 -> [Fork2PosnRawVal]
  Gain6/1 -> [Fork1PosnRawVal]
  Gain8/1 -> [Fork3PosnRawVal]
  Gain9/1 -> [Fork4PosnRawVal]
  1-D Lookup Table3/1 -> Gain37/1
  Gain37/1 -> [OddCluPRawVal]
  Gain10/1 -> [EvenCluPRawVal]
  Gain11/1 -> [ShiftSoln1IRawVal]
  Gain12/1 -> [ShiftSoln2IRawVal]
  Gain13/1 -> [MaiLineSolnIRawVal]
  Gain14/1 -> [LubeSolnIRawVal]
  Gain15/1 -> [CluSoln1IRawVal]
  Gain16/1 -> [CluSoln2IRawVal]
  [VehSpdRawVal] -> Memory1/1
  [CrnkSpdRawVal] -> Memory2/1
  [OddInpSpdRawVal] -> Memory3/1
  [EvenInpSpdRawVal] -> Memory4/1
  [OutpSpdRawVal] -> Memory5/1
  [Fork1PosnRawVal] -> Memory6/1
  [Fork2PosnRawVal] -> Memory7/1
  [Fork3PosnRawVal] -> Memory8/1
  [Fork4PosnRawVal] -> Memory9/1
  [OddCluPRawVal] -> Memory10/1
  [EvenCluPRawVal] -> Memory11/1
  Constant/1 -> Memory12/1
  Constant1/1 -> Memory13/1
  Constant2/1 -> Memory14/1
  [ShiftSoln1IRawVal] -> Memory15/1
  [ShiftSoln2IRawVal] -> Memory16/1
  [MaiLineSolnIRawVal] -> Memory17/1
  [LubeSolnIRawVal] -> Memory18/1
  [CluSoln1IRawVal] -> Memory19/1
  [CluSoln2IRawVal] -> Memory20/1
  [ShiftMux1SwtReq] -> Gain26/1
  [ShiftMux2SwtReq] -> Gain25/1
  [ShiftSoln1IReq] -> Gain24/1
  [ShiftSoln2IReq] -> Gain23/1
  [MaiLineSolnIReq] -> Gain22/1
  [LubeSolnIReq] -> Gain21/1
  [CluSoln1IReq] -> Gain20/1
  [CluSoln2IReq] -> Gain19/1
  [EngTqIntvFlg] -> Gain17/1
  [EngTqIntvRat] -> Gain18/1
  Gain17/1 -> Model/12
  Gain18/1 -> Model/11
  Gain19/1 -> Model/10
  Gain20/1 -> Model/9
  Gain21/1 -> Model/8
  Gain22/1 -> Model/7
  Gain23/1 -> Model/6
  Gain24/1 -> Model/5
  Gain25/1 -> Model/4
  Gain26/1 -> Model/3
  Gain28/1 -> Model/1
  Gain27/1 -> Model/2
  Gain29/1 -> Model/13
  [SftLvr] -> 1-D Lookup Table/1
  Gain31/1 -> Bus Creator4/1, Model1/1
  Gain30/1 -> Bus Creator4/2, Model1/2
  [throttle] -> Bus Creator3/1, [AccPedl]  "AccPedl"
  [brake] -> Gain32/1  "BrkPedl"
  [ShfLvr] -> Bus Creator3/3, [SftLvr]  "SftLvr"
  Ground/1 -> Bus Creator3/4, [Slop]  "Slop"
  [Slop] -> Gain29/1
  [BrkPedl] -> Gain27/1
  [AccPedl] -> Gain28/1
  [AccPedl] -> Gain31/1
  [BrkPedl] -> Gain30/1
  Memory2/1 -> Bus Creator4/5, Model1/5
  Memory3/1 -> Bus Creator4/6, Model1/6
  Memory4/1 -> Bus Creator4/7, Model1/7
  Memory5/1 -> Bus Creator4/8, Model1/8
  Memory6/1 -> Bus Creator4/9, Model1/9
  Memory7/1 -> Bus Creator4/10, Model1/10
  Memory8/1 -> Bus Creator4/11, Model1/11
  Memory9/1 -> Bus Creator4/12, Model1/12
  Memory10/1 -> Bus Creator4/13, Model1/13
  Memory11/1 -> Bus Creator4/14, Model1/14
  Memory12/1 -> Bus Creator4/15, Model1/15
  Memory13/1 -> Bus Creator4/16, Model1/16
  Memory14/1 -> Bus Creator4/17, Model1/17
  Memory15/1 -> Bus Creator4/18, Model1/18
  Memory16/1 -> Bus Creator4/19, Model1/19
  Memory17/1 -> Bus Creator4/20, Model1/20
  Memory18/1 -> Bus Creator4/21, Model1/21
  Memory20/1 -> Bus Creator4/23, Model1/23
  1-D Lookup Table/1 -> Bus Creator4/3, Model1/3
  Abs/1 -> Gain1/1
  Abs1/1 -> Gain2/1
  Abs2/1 -> Gain3/1
  Abs3/1 -> Gain4/1
  Abs4/1 -> Gain5/1
  Bus Creator1/1 -> Scope/3(bus3), Bus Selector1/1, Bus Selector2/1
  Bus Creator2/1 -> Scope/2(bus2)
  Model1/59 -> Bus Creator2/59, [CluSoln2Pwm]
  Model1/60 -> Bus Creator2/60, [ShiftSoln1Pwm]
  Model1/61 -> Bus Creator2/61, [ShiftSoln2Pwm]
  Model1/62 -> Bus Creator2/62, [MaiLineSolnPwm]
  Model1/58 -> Bus Creator2/58, [CluSoln1Pwm]
  Model1/63 -> Bus Creator2/63, [LubeSolnPwm]
  1-D Lookup Table1/1 -> Gain10/1
  Bus Creator3/1 -> Scope/1(bus1)
  [VehSpdTar] -> Gain38/1  "VehSpdTar"
  Gain33/1 -> 1-D Lookup Table3/1
  Gain34/1 -> 1-D Lookup Table1/1
  Model/25 -> Bus Creator1/25  "Engine Throttle [%]"
  Bus Selector2/18 -> Add/1  "<Engine Torque [Nm]>"
  Gain35/1 -> [EngTqCanVal]
  Bus Selector2/19 -> Saturation1/1  "<Engine Throttle [%]>"
  Gain36/1 -> [EngThrCanVal]
  Abs5/1 -> [EngSpdCanVal]
  [EngThrCanVal] -> Memory21/1
  Memory21/1 -> Bus Creator4/24, Model1/24
  [EngSpdCanVal] -> Memory22/1
  [EngTqCanVal] -> Memory23/1
  Memory22/1 -> Bus Creator4/25, Model1/25
  Memory23/1 -> Bus Creator4/26, Model1/26
  Model/4 -> Bus Creator1/4  "Engine Consumption Rate [g/s]"
  Add/1 -> Gain35/1
  Saturation1/1 -> Gain36/1
  Constant3/1 -> Add/2
  Memory1/1 -> Bus Creator4/4, Model1/4
  Memory19/1 -> Bus Creator4/22, Model1/22
  Bus Creator4/1 -> Scope/4(bus4)
  [ax] -> Bus Creator/4  "Ax_[ms-2]"
  [vx] -> Gain/1
  Selector1/1 -> Radians to Degrees1/1
  Selector/1 -> Radians to Degrees/1
  [PD] -> Bus Creator/10  "PDrive_[kW]"
  Radians to Degrees1/1 -> Bus Creator/12  "Pitch_[deg]"
  Radians to Degrees/1 -> Bus Creator/11  "Roll_[deg]"
  [PE] -> Bus Creator/9  "PEngine_[kW]"
  Bus Creator/1 -> Perf_Params/1
  [brake] -> Bus Creator/8  "Brake_[bar]"
  [throttle] -> Bus Creator/7  "Throttle_[perc]"
  [auto_manual] -> Bus Creator/6  "Auto_Manual_[-]"
  [ay] -> Bus Creator/5  "Ay_[ms-2]"
  [gear] -> Bus Creator/3  "Gear_[-]"
  [RPM] -> Bus Creator/2  "NEngine_[rpm]"
  Gain/1 -> Bus Creator/1  "Vx_[kmh-1]"
  Chassis/1(State) -> Selector1/1, Selector/1, State/1
  Chassis/2(VehicleSpeed_[ms-1]) -> Vx [m s-1]/1, [vx]
  Chassis/3(Vy_[ms-1]) -> [vy]
  Chassis/4(ax_[ms-2]) -> [ax]
  Chassis/5(ay_[ms-2]) -> [ay]
  Chassis/6(PDrive_[kW]) -> [PD]
  [vx] -> Bus Creator/13  "vx_[ms-1]"
  [vy] -> Bus Creator/14  "vy_[ms-1]"
  Bus Selector1/1 -> To Workspace/1  "<Engine Consumption Rate [g/s]>"
  ? -> ?

== system Traffic_Light_cs/CAR_Main/SELF_Demux ==
  SELF : Inport  OutDataTypeStr=Bus: PRESCAN_SELFSENSORDATA
  Bus Selector : BusSelector  OutputSignals=PositionX,PositionY,PositionZ,OrientationRoll,OrientationPitch,OrientationYaw,Velocity,Yaw_rate,Lat,Long,Alt
  Demux2 : Demux  Outputs=3
  Gain : Gain  Gain=180/pi
  Gain1 : Gain  Gain=180/pi
  Vector Concatenate1 : Concatenate  NumInputs=3
  compas converter : Subsystem
  x [m] : Outport
  y [m] : Outport  Port=2
  z [m] : Outport  Port=3
  rotx [deg] : Outport  Port=4
  roty [deg] : Outport  Port=5
  rotz [deg] : Outport  Port=6
  GPS lat [deg] : Outport  Port=7
  GPS long [deg] : Outport  Port=8
  GPS alt [m] : Outport  Port=9
  velocity [m/s] : Outport  Port=10
  heading [deg] : Outport  Port=11
  yaw rate [deg/s] : Outport  Port=12
  wires:
  Bus Selector/11 -> GPS alt [m]/1  "<Alt>"
  Bus Selector/10 -> GPS long [deg]/1  "<Long>"
  Bus Selector/9 -> GPS lat [deg]/1  "<Lat>"
  Bus Selector/8 -> Gain1/1  "<Yaw_rate>"
  Bus Selector/7 -> velocity [m/s]/1  "<Velocity>"
  Bus Selector/6 -> compas converter/1(rotz [rad]), Vector Concatenate1/3  "<OrientationYaw>"
  Bus Selector/5 -> Vector Concatenate1/2  "<OrientationPitch>"
  Bus Selector/4 -> Vector Concatenate1/1  "<OrientationRoll>"
  Vector Concatenate1/1 -> Gain/1
  Bus Selector/3 -> z [m]/1  "<PositionZ>"
  Bus Selector/2 -> y [m]/1  "<PositionY>"
  Bus Selector/1 -> x [m]/1  "<PositionX>"
  SELF/1 -> Bus Selector/1
  Gain/1 -> Demux2/1
  Demux2/1 -> rotx [deg]/1
  Demux2/2 -> roty [deg]/1
  Demux2/3 -> rotz [deg]/1
  compas converter/1(heading [deg]) -> heading [deg]/1
  Gain1/1 -> yaw rate [deg/s]/1

== system Traffic_Light_cs/CAR_Main/STATE_CAR_Main ==
  State : Inport  SampleTime=TimeStep
  Bus Creator : BusCreator  Inputs=15  OutDataTypeStr=Bus: PRESCAN_STATEACTUATORDATA  NonVirtualBus=on
  Demux : Demux  Outputs=15
  iniBODYAngles wrtVEH [rad] : Constant  Value=[Roll0 Pitch0 0]  SampleTime=TimeStep
  iniVEHAngles wrtGLOB [rad] : Constant  Value=[0 0 Yaw0]  SampleTime=TimeStep
  iniVEHposition wrtGLOB [m] : Constant  Value=[x0 y0 z0]  SampleTime=TimeStep
  state2FullState : PreScanSimulinkLibrary/state2FullState  SystemSampleTime=-1  Latency=0  AutoFrameSizeCalculation=off
  StateBus : Outport  OutDataTypeStr=Bus: PRESCAN_STATEACTUATORDATA
  wires:
  Bus Creator/1 -> StateBus/1
  State/1 -> state2FullState/1
  state2FullState/1 -> Demux/1
  iniVEHposition wrtGLOB [m]/1 -> state2FullState/2
  iniBODYAngles wrtVEH [rad]/1 -> state2FullState/3
  iniVEHAngles wrtGLOB [rad]/1 -> state2FullState/4
  Demux/1 -> Bus Creator/1  "PositionX"
  Demux/2 -> Bus Creator/2  "PositionY"
  Demux/3 -> Bus Creator/3  "PositionZ"
  Demux/4 -> Bus Creator/4  "VelocityX"
  Demux/5 -> Bus Creator/5  "VelocityY"
  Demux/6 -> Bus Creator/6  "VelocityZ"
  Demux/7 -> Bus Creator/7  "AccelerationX"
  Demux/8 -> Bus Creator/8  "AccelerationY"
  Demux/9 -> Bus Creator/9  "AccelerationZ"
  Demux/10 -> Bus Creator/10  "OrientationRoll"
  Demux/11 -> Bus Creator/11  "OrientationPitch"
  Demux/12 -> Bus Creator/12  "OrientationYaw"
  Demux/13 -> Bus Creator/13  "AngularVelocityRoll"
  Demux/14 -> Bus Creator/14  "AngularVelocityPitch"
  Demux/15 -> Bus Creator/15  "AngularVelocityYaw"

== system Traffic_Light_cs/CAR_Main/Subsystem1 ==
  light_time : Inport
  light_type : Inport  Port=2
  distance : Inport  Port=3
  speed : Inport  Port=4
  Divide : Product  Inputs=*/
  Divide1 : Product  Inputs=/*
  Fuzzy Logic Controller : fuzblock/Fuzzy Logic  Controller  FIS='y.fis'  OutputSampleNumber=101  DataType=double  FuzzifiedInputs=off  RuleFiringStrengths=off  RuleOutputs=off  AggregatedOutputs=off  SimulateUsing=Interpreted execution  OutOfRangeInputValueMessage=warning  NoRuleFiredMessage=warning  EmptyOutputFuzzySetMessage=warning
  Subsystem : Subsystem
  Out1 : Outport  VectorParamsAs1DForOutWhenUnconnected=off
  wires:
  distance/1 -> Divide/1
  Fuzzy Logic Controller/1 -> Out1/1
  Subsystem/1(Out2) -> Divide1/1
  light_time/1 -> Subsystem/1(light_time)
  Divide1/1 -> Fuzzy Logic Controller/1
  light_type/1 -> Subsystem/2(light_type)
  speed/1 -> Divide/2
  Divide/1 -> Divide1/2

== system Traffic_Light_cs/CAR_Main/V2V_Input ==
  TrafficLight_ID_Main : Inport
  Light_Information1 : Inport  Tag=inport/SelfPort  Port=2  PortDimensions=3  SampleTime=1/20  BusOutputAsStruct=on
  Bus Selector1 : BusSelector  OutputSignals=ID_Ahead,LightState_Ahead,TrafficTime_Ahead
  Chart1 : Stateflow chart  TreatAsAtomicUnit=on
  Chart2 : Stateflow chart  Priority=2  TreatAsAtomicUnit=on
  MATLAB Function : MATLAB Function  Priority=1  TreatAsAtomicUnit=on
  Memory : Memory
  Memory1 : Memory
  Memory2 : Memory
  Traffic_State : Outport  VectorParamsAs1DForOutWhenUnconnected=off
  Traffic_Time : Outport  Port=2  VectorParamsAs1DForOutWhenUnconnected=off
  wires:
  Chart1/2(time) -> Traffic_Time/1
  [now_time] -> Chart1/3(now_time)
  MATLAB Function/2(Traffic_now_Time) -> [now_time]  "now_time_Main"
  [State_Next] -> Memory1/1
  [next_time] -> Chart2/3(next_time)
  Chart2/3(localnextID) -> [TrafficID_Next]
  Bus Selector1/2 -> MATLAB Function/3(Light_State_Ahead)  "<LightState_Ahead>"
  TrafficLight_ID_Main/1 -> MATLAB Function/1(Traffic_ID), Chart1/1(TrafficID), Chart2/1(TrafficID)
  [Time_Next] -> Memory2/1
  [now_state] -> Chart1/2(now_state)
  Chart2/1(state) -> [State_Next]
  Bus Selector1/1 -> MATLAB Function/2(TrafficLight_ID_Ahead)  "<ID_Ahead>"
  MATLAB Function/1(Traffic_now_State) -> [now_state]  "now_state_Main"
  MATLAB Function/4(Traffic_next_Time) -> [next_time]  "next_time_Main"
  Bus Selector1/3 -> MATLAB Function/4(Traffic_Time1)  "<TrafficTime_Ahead>"
  Chart1/1(state) -> Traffic_State/1
  Memory2/1 -> MATLAB Function/7(Time_Next)
  Memory/1 -> MATLAB Function/5(TrafficID_Next)
  Memory1/1 -> MATLAB Function/6(State_Next)
  [TrafficID_Next] -> Memory/1
  [next_state] -> Chart2/2(next_state)
  Chart2/2(time) -> [Time_Next]
  MATLAB Function/3(Traffic_next_State) -> [next_state]  "next_state_Main"
  Light_Information1/1 -> Bus Selector1/1

== system Traffic_Light_cs/CAR_Main/V2V_Output ==
  Traffic_State : Inport
  Dis_Car2Light_Main : Inport  Port=2
  Light_State_Main : Inport  Port=3
  TrafficLight_ID_Main : Inport  Port=4
  Traffic_Time : Inport  Port=5
  TrafficLight_PhaseTime : Inport  Port=6
  Bus Creator : BusCreator  Inputs=3
  Switch : Switch  Criteria=u2 > Threshold
  Switch1 : Switch  Criteria=u2 > Threshold  Threshold=500
  Traffic_Information : Outport  VectorParamsAs1DForOutWhenUnconnected=off
  "Traffic_Time " : Outport  Port=2  VectorParamsAs1DForOutWhenUnconnected=off
  wires:
  Light_State_Main/1 -> Switch1/3
  Bus Creator/1 -> Traffic_Information/1
  Traffic_State/1 -> Switch1/1
  TrafficLight_PhaseTime/1 -> Switch/3
  Switch1/1 -> Bus Creator/1  "LightState_Main"
  TrafficLight_ID_Main/1 -> Bus Creator/2  "ID_Main"
  Traffic_Time/1 -> Switch/1, Switch/2
  Dis_Car2Light_Main/1 -> Switch1/2
  Switch/1 -> Bus Creator/3, "Traffic_Time "/1  "TrafficTime_Main"

== system Traffic_Light_cs/CAR_Main/pre ==
  x [m] : Inport
  y [m] : Inport  Port=2
  Subsystem : Subsystem
  Subsystem1 : Subsystem
  Subsystem2 : Subsystem
  Dis_Car2Light_Main : Outport
  TrafficLight_ID_Main : Outport  Port=2
  angle : Outport  Port=3
  grade : Outport  Port=4
  wires:
  Subsystem/1(Distance2Light) -> Dis_Car2Light_Main/1  "Dis_Car2Light_Main"
  Subsystem2/1(angle) -> angle/1  "angle"
  Subsystem/2(TrafficLight_ID) -> TrafficLight_ID_Main/1  "TrafficLight_ID_Main"
  y [m]/1 -> Subsystem1/2(Car_Y), Subsystem2/2(Car_Y), Subsystem/2(y [m])
  x [m]/1 -> Subsystem1/1(Car_X), Subsystem2/1(Car_X), Subsystem/1(x [m])
  Subsystem1/1(grade) -> grade/1  "grade"

== system Traffic_Light_cs/ID_1/Subsystem ==
  Green : Inport
  Yellow : Inport  Port=2
  Red : Inport  Port=3
  MATLAB Function : MATLAB Function  TreatAsAtomicUnit=on
  Out1 : Outport
  wires:
  Green/1 -> MATLAB Function/1(green)
  Yellow/1 -> MATLAB Function/2(yellow)
  Red/1 -> MATLAB Function/3(rad)
  MATLAB Function/1(state) -> Out1/1

== system Traffic_Light_cs/ID_1/VISUCasingLights_Mux ==
  Green [-] : Inport  Tag=inport/Green [-]  SampleTime=1/1000  BusOutputAsStruct=on
  Orange [-] : Inport  Tag=inport/Orange [-]  Port=2  SampleTime=1/1000  BusOutputAsStruct=on
  Red [-] : Inport  Tag=inport/Red [-]  Port=3  SampleTime=1/1000  BusOutputAsStruct=on
  MuxVisuLights : Mux  Inputs=3
  VISUCasingLights_ID_1 : Outport  Tag=outport/VisuCasingLights  SampleTime=1/1000
  wires:
  MuxVisuLights/1 -> VISUCasingLights_ID_1/1
  Green [-]/1 -> MuxVisuLights/1
  Orange [-]/1 -> MuxVisuLights/2
  Red [-]/1 -> MuxVisuLights/3

== system Traffic_Light_cs/ID_2/Subsystem ==
  Green : Inport
  Yellow : Inport  Port=2
  Red : Inport  Port=3
  MATLAB Function : MATLAB Function  TreatAsAtomicUnit=on
  Out1 : Outport
  wires:
  Green/1 -> MATLAB Function/1(green)
  Yellow/1 -> MATLAB Function/2(yellow)
  Red/1 -> MATLAB Function/3(rad)
  MATLAB Function/1(state) -> Out1/1

== system Traffic_Light_cs/ID_2/VISUCasingLights_Mux ==
  Green [-] : Inport  Tag=inport/Green [-]  SampleTime=1/1000  BusOutputAsStruct=on
  Orange [-] : Inport  Tag=inport/Orange [-]  Port=2  SampleTime=1/1000  BusOutputAsStruct=on
  Red [-] : Inport  Tag=inport/Red [-]  Port=3  SampleTime=1/1000  BusOutputAsStruct=on
  MuxVisuLights : Mux  Inputs=3
  VISUCasingLights_ID_2 : Outport  Tag=outport/VisuCasingLights  SampleTime=1/1000
  wires:
  MuxVisuLights/1 -> VISUCasingLights_ID_2/1
  Green [-]/1 -> MuxVisuLights/1
  Orange [-]/1 -> MuxVisuLights/2
  Red [-]/1 -> MuxVisuLights/3

== system Traffic_Light_cs/ID_3/Subsystem ==
  Green : Inport
  Yellow : Inport  Port=2
  Red : Inport  Port=3
  MATLAB Function : MATLAB Function  TreatAsAtomicUnit=on
  Out1 : Outport
  wires:
  Green/1 -> MATLAB Function/1(green)
  Yellow/1 -> MATLAB Function/2(yellow)
  Red/1 -> MATLAB Function/3(rad)
  MATLAB Function/1(state) -> Out1/1

== system Traffic_Light_cs/ID_3/VISUCasingLights_Mux ==
  Green [-] : Inport  Tag=inport/Green [-]  SampleTime=1/1000  BusOutputAsStruct=on
  Orange [-] : Inport  Tag=inport/Orange [-]  Port=2  SampleTime=1/1000  BusOutputAsStruct=on
  Red [-] : Inport  Tag=inport/Red [-]  Port=3  SampleTime=1/1000  BusOutputAsStruct=on
  MuxVisuLights : Mux  Inputs=3
  VISUCasingLights_ID_3 : Outport  Tag=outport/VisuCasingLights  SampleTime=1/1000
  wires:
  MuxVisuLights/1 -> VISUCasingLights_ID_3/1
  Green [-]/1 -> MuxVisuLights/1
  Orange [-]/1 -> MuxVisuLights/2
  Red [-]/1 -> MuxVisuLights/3
